simulink model "VSG"  (R2022a)
settings: Solver=ode23t  StartTime=0.0  StopTime=3  RelTol=1e-3
values from neighbouring files (symbols this model uses):
  C = 5600e-6    (= 0.0056)    [param.m]
  Cf = 35e-6    (= 3.5e-05)    [param.m]
  D = 3.24e4/w0    (= 103.132403124)    [param.m]
  E0 = 311    [param.m]
  fn = 50    [param.m]
  Ib = Sb/(sqrt(3)*Ub)    [param.m]
  J = 3.36    [param.m]
  Kf = 0.95e4/w0    (= 30.2394391875)    [param.m]
  Ki = 0.5*sqrt(3)*Sb/Ub    [param.m]
  Kq = (2500*6000)/(800e3*sqrt(3))    [param.m]
  L = 3e-3    (= 0.003)    [param.m]
  Pref = 170e3    (= 170000)    [param.m]
  R = 0.5    [param.m]
  Rc = 1e-3    (= 0.001)    [param.m]
  Rf = 0.05    [param.m]
  Sb = 800e3    (= 800000)    [param.m]
  Ts = 1/20e3    (= 5e-05)    [param.m]
  Ub = 6e3    (= 6000)    [param.m]
  Un = 380    [param.m]
  w0 = 2*pi*fn    (= 314.159265359)    [param.m]
libraries: spsIGBTDiodeLib x14, spsSeriesRLCBranchLib x9, slpidlib x7, spsDiodeLib x6, spsVoltageMeasurementLib x6, spsabctodq0Lib x4, spsThreePhaseVIMeasurementLib x3, eePowerMeasurement x2, simulink x2, spsDCVoltageSourceLib x1, spsGroundLib x1, spsPower3phInstantaneousLib x1
(part 2 of 2)

== matlab function VSG/SVPWM调制/SVPWM/下半周期时间分配 ==
  data: TA input; TB input; TC input; n input; t1 output; t2 output; t3 output
function [t1,t2,t3] = TimeShare(TA,TB,TC,n)

t1=0;
t2=0;
t3=0;

if (n==1)
    t1 = TC;
    t2 = TB;
    t3 = TA;
end

if (n==2)
    t1 = TA;
    t2 = TC;
    t3 = TB;
end

if (n==3)
    t1 = TA;
    t2 = TB;
    t3 = TC;
end

if (n==4)
    t1 = TC;
    t2 = TA;
    t3 = TB;
end

if (n==5)
    t1 = TB;
    t2 = TA;
    t3 = TC;
end

if (n==6)
    t1 = TB;
    t2 = TA;
    t3 = TC;
end

== matlab function VSG/SVPWM调制/SVPWM/按规律选择实际时间分配 ==
  data: ta1 input; tb1 input; tc1 input; ta2 input; T1 output; T2 output; T3 output; tb2 input; tc2 input; N input
function [T1,T2,T3] = SwitchTime(ta1,tb1,tc1,ta2,tb2,tc2,N)
T1 = 0;
T2 = 0;
T3 = 0;
if (N == 1)
    T1 = ta1;
    T2 = tb1;
    T3 = tc1;
end

if (N == 2)
    T1 = ta2;
    T2 = tb2;
    T3 = tc2;
end

if (N == 3)
    T1 = ta1;
    T2 = tb1;
    T3 = tc1;
end

if (N == 4)
    T1 = ta2;
    T2 = tb2;
    T3 = tc2;
end

if (N == 5)
    T1 = ta1;
    T2 = tb1;
    T3 = tc1;
end

if (N == 6)
    T1 = ta2;
    T2 = tb2;
    T3 = tc2;
end

== matlab function VSG/SVPWM调制/SVPWM/第一大扇区羊角分配 ==
  data: n input; T1 input; T2 input; T3 input; t11 output; t21 output; t31 output
function [t11,t21,t31] = VectorShare(n,T1,T2,T3)
t11 = 0;
t21 = 0;
t31 = 0;
if (n==1)
    t11 = T1/2;
    t21 = -T1/2;
    t31 = -T1/2-T2;
end
if (n==2)
    t11 = T1/2+T3;
    t21 = T1/2;
    t31 = -T1/2;
end
if (n==3)
    t11 = T1/2+T3;
    t21 = -T1/2;
    t31 = -T1/2-T2-T3;
end
if (n==4)
    t11 = T1/2+T2+T3;
    t21 = T1/2;
    t31 = -T1/2-T2;
end
if (n==5)
    t11 = T1/2+T2+T3;
    t21 = -T1/2-T2;
    t31 = -T1/2-T2-T3;
end
if (n==6)
    t11 = T1/2+T2+T3;
    t21 = T1/2+T3;
    t31 = -T1/2-T2-T3;
end
